simulink model "balance_bike"  (R2025a)
settings: Solver=ode45  StartTime=0.0  StopTime=50  MaxStep=0.0001  RelTol=1e-6
values from neighbouring files (symbols this model uses):
  angle_Kp = 7.5    [init_balance_bike.m]
  angle_out_max = 2000    [init_balance_bike.m]
  fly_mech_den = [J_total, B_fly]    [init_balance_bike.m]
  fly_mech_num = [1]    [init_balance_bike.m]
  gyro_Kp = 26.5    [init_balance_bike.m]
  gyro_out_max = 2000    [init_balance_bike.m]
  J_body = m_body * h_body^2    (= 0.0675)    [init_balance_bike.m]
  K_enc = PPR * Ts / (2*pi)    (= 3.18309886184)    [init_balance_bike.m]
  Ke = 0.08    [init_balance_bike.m]
  Kt = 0.08    [init_balance_bike.m]
  mgh = m_body * g * h_body    (= 4.4145)    [init_balance_bike.m]
  motor_elec_den = [La, Ra]    [init_balance_bike.m]
  motor_elec_num = [1]    [init_balance_bike.m]
  PWM_to_V = V_supply / 2000    (= 0.006)    [init_balance_bike.m]
  vel_integral_max = 500    [init_balance_bike.m]
  vel_Kd_cont = 0.015 * Ts    (= 7.5e-05)    [init_balance_bike.m]
  vel_Ki_cont = 0.000045 / Ts    (= 0.009)    [init_balance_bike.m]
  vel_Kp = 0.065    [init_balance_bike.m]
  vel_out_max = 2000    [init_balance_bike.m]
libraries: slpidlib x3
settings Model: Creator=apple  LastModifiedBy=apple

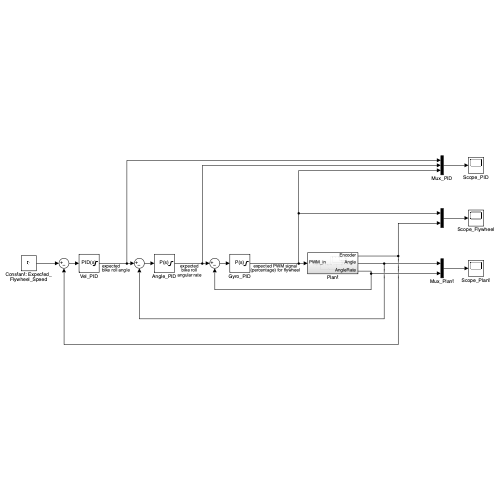
[thumbnail: Simulink's stored preview of the top-level diagram]
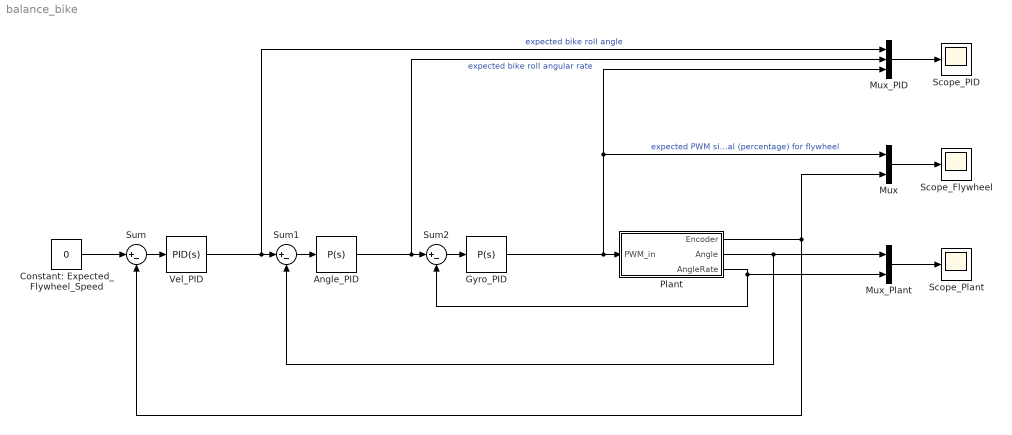
== system balance_bike ==
  Angle_PID : slpidlib/PID Controller  Controller=P  Form=Parallel  TimeDomain=Continuous-time  UseExternalTs=off  SampleTime=-1  IntegratorMethod=Forward Euler  FilterMethod=Forward Euler  ControllerParametersSource=internal  P=angle_Kp  I=1  UseKiTs=off  D=0  UseExternalDerivativeSource=off  N=100  UseFilter=on  TunerSelectOption=Transfer Function Based (PID Tuner App)  InitialConditionSource=internal  InitialConditionForIntegrator=0  InitialConditionForFilter=0  DifferentiatorICPrevScaledInput=0  ExternalReset=none  TrackingMode=off  Kt=1  LimitOutput=on  SatLimitsSource=internal  UpperSaturationLimit=angle_out_max  LowerSaturationLimit=-angle_out_max  LinearizeAsGain=on  AntiWindupMode=none  Kb=1  LimitIntegrator=off  UpperIntegratorSaturationLimit=inf  LowerIntegratorSaturationLimit=-inf  POutMin=[]  POutMax=[]  IOutMin=[]  IOutMax=[]  DOutMin=[]  DOutMax=[]  NOutMin=[]  NOutMax=[]  SumOutMin=[]  SumOutMax=[]  SaturationOutMin=[]  SaturationOutMax=[]  PParamMin=[]  PParamMax=[]  IParamMin=[]  IParamMax=[]  DParamMin=[]  DParamMax=[]  NParamMin=[]  NParamMax=[]  KbParamMin=[]  KbParamMax=[]  KtParamMin=[]  KtParamMax=[]  KbOutMin=[]  KbOutMax=[]  KtOutMin=[]  KtOutMax=[]  IntegratorOutMin=[]  IntegratorOutMax=[]  FilterOutMin=[]  FilterOutMax=[]  SumI1OutMin=[]  SumI1OutMax=[]  SumI2OutMin=[]  SumI2OutMax=[]  SumI3OutMin=[]  SumI3OutMax=[]  SumI4OutMin=[]  SumI4OutMax=[]  SumDOutMin=[]  SumDOutMax=[]  DifferentiatorOutMin=[]  DifferentiatorOutMax=[]  FilterDiffOutCoefMin=[]  FilterDiffOutCoefMax=[]  ReciprocalOutMin=[]  ReciprocalOutMax=[]  SumDenOutMin=[]  SumDenOutMax=[]  SumNumOutMin=[]  SumNumOutMax=[]  DivideOutMin=[]  DivideOutMax=[]  UdiffTsProdOutMin=[]  UdiffTsProdOutMax=[]  NTsProdOutMin=[]  NTsProdOutMax=[]  UintegralTsProdOutMin=[]  UintegralTsProdOutMax=[]  UngainTsProdOutMin=[]  UngainTsProdOutMax=[]  ClampingZeroOutDataTypeStr=Inherit: Inherit via back propagation  ClampingZeroOutMin=[]  ClampingZeroOutMax=[]  FilterDenConstantOutDataTypeStr=Inherit: Inherit via back propagation  FilterDenConstantOutMin=[]  FilterDenConstantOutMax=[]  PCopyOutDataTypeStr=Inherit: Inherit via back propagation  PCopyOutMin=[]  PCopyOutMax=[]  NCopyOutDataTypeStr=Inherit: Inherit via back propagation  NCopyOutMin=[]  NCopyOutMax=[]  IntegratorContinuousStateAttributes=''  IntegratorStateMustResolveToSignalObject=off  IntegratorRTWStateStorageClass=Auto  FilterContinuousStateAttributes=''  FilterStateMustResolveToSignalObject=off  FilterRTWStateStorageClass=Auto  ParallelPVariant=InternalParameters  IdealPVariant=Disabled  IVariant=Disabled  DVariant=Disabled  IntegratorVariant=Disabled  SatVariant=Enabled  AWVariant=Disabled  PCopyVariant=Disabled  TRVariant=Disabled  FdbkBlocksVariant=Forward  IdealPFdbkVariant=Disabled  SatFdbkVariant=Disabled  DerivativeFilterVariant=Disabled  NVariant=Disabled  NCopyVariant=Disabled_SignalSpec  FilterICVariant=Disabled  IntegratorICVariant=Disabled  ExternalResetVariant=Disabled  TRSumVariant=Passthrough  SumFdbkVariant=Disabled  SumVariant=Passthrough_P  TsampFilterVariant=InternalTs  TsampNgainVariant=Passthrough  TsampIntegralVariant=Disabled_SignalSpec  ExternalSaturationOutDataTypeStr=Inherit: Same as second input  DerivativeSourceVariant=Disabled  PreIntVariant=InternalPreInt
  Constant: Expected_ Flywheel_Speed : Constant  Value=0
  Gyro_PID : slpidlib/PID Controller  Controller=P  Form=Parallel  TimeDomain=Continuous-time  UseExternalTs=off  SampleTime=-1  IntegratorMethod=Forward Euler  FilterMethod=Forward Euler  ControllerParametersSource=internal  P=gyro_Kp  I=1  UseKiTs=off  D=0  UseExternalDerivativeSource=off  N=100  UseFilter=on  TunerSelectOption=Transfer Function Based (PID Tuner App)  InitialConditionSource=internal  InitialConditionForIntegrator=0  InitialConditionForFilter=0  DifferentiatorICPrevScaledInput=0  ExternalReset=none  TrackingMode=off  Kt=1  LimitOutput=on  SatLimitsSource=internal  UpperSaturationLimit=gyro_out_max  LowerSaturationLimit=-gyro_out_max  LinearizeAsGain=on  AntiWindupMode=none  Kb=1  LimitIntegrator=off  UpperIntegratorSaturationLimit=inf  LowerIntegratorSaturationLimit=-inf  POutMin=[]  POutMax=[]  IOutMin=[]  IOutMax=[]  DOutMin=[]  DOutMax=[]  NOutMin=[]  NOutMax=[]  SumOutMin=[]  SumOutMax=[]  SaturationOutMin=[]  SaturationOutMax=[]  PParamMin=[]  PParamMax=[]  IParamMin=[]  IParamMax=[]  DParamMin=[]  DParamMax=[]  NParamMin=[]  NParamMax=[]  KbParamMin=[]  KbParamMax=[]  KtParamMin=[]  KtParamMax=[]  KbOutMin=[]  KbOutMax=[]  KtOutMin=[]  KtOutMax=[]  IntegratorOutMin=[]  IntegratorOutMax=[]  FilterOutMin=[]  FilterOutMax=[]  SumI1OutMin=[]  SumI1OutMax=[]  SumI2OutMin=[]  SumI2OutMax=[]  SumI3OutMin=[]  SumI3OutMax=[]  SumI4OutMin=[]  SumI4OutMax=[]  SumDOutMin=[]  SumDOutMax=[]  DifferentiatorOutMin=[]  DifferentiatorOutMax=[]  FilterDiffOutCoefMin=[]  FilterDiffOutCoefMax=[]  ReciprocalOutMin=[]  ReciprocalOutMax=[]  SumDenOutMin=[]  SumDenOutMax=[]  SumNumOutMin=[]  SumNumOutMax=[]  DivideOutMin=[]  DivideOutMax=[]  UdiffTsProdOutMin=[]  UdiffTsProdOutMax=[]  NTsProdOutMin=[]  NTsProdOutMax=[]  UintegralTsProdOutMin=[]  UintegralTsProdOutMax=[]  UngainTsProdOutMin=[]  UngainTsProdOutMax=[]  ClampingZeroOutDataTypeStr=Inherit: Inherit via back propagation  ClampingZeroOutMin=[]  ClampingZeroOutMax=[]  FilterDenConstantOutDataTypeStr=Inherit: Inherit via back propagation  FilterDenConstantOutMin=[]  FilterDenConstantOutMax=[]  PCopyOutDataTypeStr=Inherit: Inherit via back propagation  PCopyOutMin=[]  PCopyOutMax=[]  NCopyOutDataTypeStr=Inherit: Inherit via back propagation  NCopyOutMin=[]  NCopyOutMax=[]  IntegratorContinuousStateAttributes=''  IntegratorStateMustResolveToSignalObject=off  IntegratorRTWStateStorageClass=Auto  FilterContinuousStateAttributes=''  FilterStateMustResolveToSignalObject=off  FilterRTWStateStorageClass=Auto  ParallelPVariant=InternalParameters  IdealPVariant=Disabled  IVariant=Disabled  DVariant=Disabled  IntegratorVariant=Disabled  SatVariant=Enabled  AWVariant=Disabled  PCopyVariant=Disabled  TRVariant=Disabled  FdbkBlocksVariant=Forward  IdealPFdbkVariant=Disabled  SatFdbkVariant=Disabled  DerivativeFilterVariant=Disabled  NVariant=Disabled  NCopyVariant=Disabled_SignalSpec  FilterICVariant=Disabled  IntegratorICVariant=Disabled  ExternalResetVariant=Disabled  TRSumVariant=Passthrough  SumFdbkVariant=Disabled  SumVariant=Passthrough_P  TsampFilterVariant=InternalTs  TsampNgainVariant=Passthrough  TsampIntegralVariant=Disabled_SignalSpec  ExternalSaturationOutDataTypeStr=Inherit: Same as second input  DerivativeSourceVariant=Disabled  PreIntVariant=InternalPreInt
  Mux : Mux  Inputs=2
  Mux_PID : Mux  Inputs=3
  Mux_Plant : Mux  Inputs=2
  Plant : Subsystem
  Scope_Flywheel : Scope
      settings: ActiveDisplayYMinimum=-2400.6327849679374  ActiveDisplayYMaximum=1605.6950647114356  DataLoggingVariableName=ScopeData3
  Scope_PID : Scope
      settings: ActiveDisplayYMinimum=-154.84030176969517  ActiveDisplayYMaximum=142.23646338458198
  Scope_Plant : Scope
      settings: ActiveDisplayYMinimum=-271.32237156661733  ActiveDisplayYMaximum=384.67484580037069  DataLoggingVariableName=ScopeData2
  Sum : Sum  Inputs=|+-
  Sum1 : Sum  Inputs=|+-
  Sum2 : Sum  Inputs=|+-
  Vel_PID : slpidlib/PID Controller  Controller=PID  Form=Parallel  TimeDomain=Continuous-time  UseExternalTs=off  SampleTime=-1  IntegratorMethod=Forward Euler  FilterMethod=Forward Euler  ControllerParametersSource=internal  P=vel_Kp  I=vel_Ki_cont  UseKiTs=off  D=vel_Kd_cont  UseExternalDerivativeSource=off  N=100  UseFilter=on  TunerSelectOption=Transfer Function Based (PID Tuner App)  InitialConditionSource=internal  InitialConditionForIntegrator=0  InitialConditionForFilter=0  DifferentiatorICPrevScaledInput=0  ExternalReset=none  TrackingMode=off  Kt=1  LimitOutput=on  SatLimitsSource=internal  UpperSaturationLimit=vel_out_max  LowerSaturationLimit=-vel_out_max  LinearizeAsGain=on  AntiWindupMode=none  Kb=1  LimitIntegrator=on  UpperIntegratorSaturationLimit=vel_integral_max  LowerIntegratorSaturationLimit=-vel_integral_max  POutMin=[]  POutMax=[]  IOutMin=[]  IOutMax=[]  DOutMin=[]  DOutMax=[]  NOutMin=[]  NOutMax=[]  SumOutMin=[]  SumOutMax=[]  SaturationOutMin=[]  SaturationOutMax=[]  PParamMin=[]  PParamMax=[]  IParamMin=[]  IParamMax=[]  DParamMin=[]  DParamMax=[]  NParamMin=[]  NParamMax=[]  KbParamMin=[]  KbParamMax=[]  KtParamMin=[]  KtParamMax=[]  KbOutMin=[]  KbOutMax=[]  KtOutMin=[]  KtOutMax=[]  IntegratorOutMin=[]  IntegratorOutMax=[]  FilterOutMin=[]  FilterOutMax=[]  SumI1OutMin=[]  SumI1OutMax=[]  SumI2OutMin=[]  SumI2OutMax=[]  SumI3OutMin=[]  SumI3OutMax=[]  SumI4OutMin=[]  SumI4OutMax=[]  SumDOutMin=[]  SumDOutMax=[]  DifferentiatorOutMin=[]  DifferentiatorOutMax=[]  FilterDiffOutCoefMin=[]  FilterDiffOutCoefMax=[]  ReciprocalOutMin=[]  ReciprocalOutMax=[]  SumDenOutMin=[]  SumDenOutMax=[]  SumNumOutMin=[]  SumNumOutMax=[]  DivideOutMin=[]  DivideOutMax=[]  UdiffTsProdOutMin=[]  UdiffTsProdOutMax=[]  NTsProdOutMin=[]  NTsProdOutMax=[]  UintegralTsProdOutMin=[]  UintegralTsProdOutMax=[]  UngainTsProdOutMin=[]  UngainTsProdOutMax=[]  ClampingZeroOutDataTypeStr=Inherit: Inherit via back propagation  ClampingZeroOutMin=[]  ClampingZeroOutMax=[]  FilterDenConstantOutDataTypeStr=Inherit: Inherit via back propagation  FilterDenConstantOutMin=[]  FilterDenConstantOutMax=[]  PCopyOutDataTypeStr=Inherit: Inherit via back propagation  PCopyOutMin=[]  PCopyOutMax=[]  NCopyOutDataTypeStr=Inherit: Inherit via back propagation  NCopyOutMin=[]  NCopyOutMax=[]  IntegratorContinuousStateAttributes=''  IntegratorStateMustResolveToSignalObject=off  IntegratorRTWStateStorageClass=Auto  FilterContinuousStateAttributes=''  FilterStateMustResolveToSignalObject=off  FilterRTWStateStorageClass=Auto  ParallelPVariant=InternalParameters  IdealPVariant=Disabled  IVariant=InternalParameters  DVariant=InternalParameters  IntegratorVariant=Continuous  SatVariant=Enabled  AWVariant=Passthrough  PCopyVariant=Disabled  TRVariant=Disabled  FdbkBlocksVariant=Forward  IdealPFdbkVariant=Disabled  SatFdbkVariant=Disabled  DerivativeFilterVariant=ContFilter  NVariant=InternalParameters  NCopyVariant=Disabled  FilterICVariant=InternalICsFilter  IntegratorICVariant=InternalICs  ExternalResetVariant=Disabled  TRSumVariant=Passthrough  SumFdbkVariant=Disabled  SumVariant=Sum_PID  TsampFilterVariant=InternalTs  TsampNgainVariant=Passthrough  TsampIntegralVariant=Disabled_SignalSpec  ExternalSaturationOutDataTypeStr=Inherit: Same as second input  DerivativeSourceVariant=ErrorSignal  PreIntVariant=InternalPreInt
  wires:
  Plant/1(Encoder) -> Mux/2, Sum/2
  Plant/3(AngleRate) -> Mux_Plant/2, Sum2/2
  Plant/2(Angle) -> Sum1/2, Mux_Plant/1
  Constant: Expected_ Flywheel_Speed/1 -> Sum/1
  Sum1/1 -> Angle_PID/1
  Sum2/1 -> Gyro_PID/1
  Angle_PID/1 -> Mux_PID/2, Sum2/1  "expected bike roll angular rate"
  Sum/1 -> Vel_PID/1
  Gyro_PID/1 -> Mux/1, Mux_PID/3, Plant/1(PWM_in)  "expected PWM signal (percentage) for flywheel"
  Mux_PID/1 -> Scope_PID/1
  Mux_Plant/1 -> Scope_Plant/1
  Vel_PID/1 -> Mux_PID/1, Sum1/1  "expected bike roll angle"
  Mux/1 -> Scope_Flywheel/1

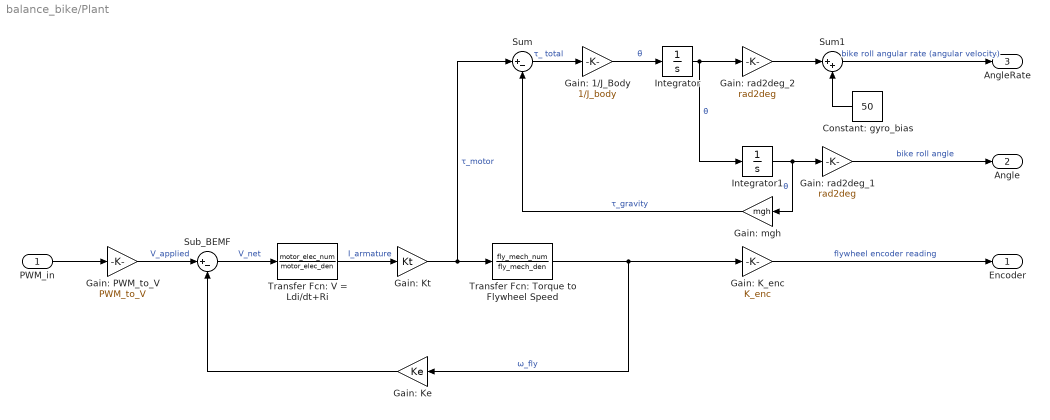
== system balance_bike/Plant ==
  PWM_in : Inport
  Constant: gyro_bias : Constant  Value=50
  Gain: 1/J_Body : Gain  Gain=1/J_body
  Gain: K_enc : Gain  Gain=K_enc
  Gain: Ke : Gain  Gain=Ke
  Gain: Kt : Gain  Gain=Kt
  Gain: PWM_to_V : Gain  Gain=PWM_to_V
  Gain: mgh : Gain  Gain=mgh
  Gain: rad2deg_1 : Gain  Gain=rad2deg
  Gain: rad2deg_2 : Gain  Gain=rad2deg
  Integrator : Integrator
  Integrator1 : Integrator  InitialCondition=0.5
  Sub_BEMF : Sum  Inputs=|+-
  Sum : Sum  Inputs=|+-
  Sum1 : Sum  Inputs=|++
  Transfer Fcn: V = Ldi/dt+Ri : TransferFcn  Numerator=motor_elec_num  Denominator=motor_elec_den
  Transfer Fcn: Torque to Flywheel Speed : TransferFcn  Numerator=fly_mech_num  Denominator=fly_mech_den
  Encoder : Outport
  Angle : Outport  Port=2
  AngleRate : Outport  Port=3
  wires:
  Gain: mgh/1 -> Sum/2  "τ_gravity"
  Gain: PWM_to_V/1 -> Sub_BEMF/1  "V_applied"
  Transfer Fcn: V = Ldi/dt+Ri/1 -> Gain: Kt/1  "I_armature"
  Integrator/1 -> Gain: rad2deg_2/1, Integrator1/1  "θ̇"
  Gain: rad2deg_2/1 -> Sum1/1
  Gain: rad2deg_1/1 -> Angle/1  "bike roll angle"
  Sum/1 -> Gain: 1/J_Body/1  "τ_ total"
  Gain: 1/J_Body/1 -> Integrator/1  "θ̈"
  Integrator1/1 -> Gain: rad2deg_1/1, Gain: mgh/1  "θ"
  Constant: gyro_bias/1 -> Sum1/2
  Gain: Kt/1 -> Sum/1, Transfer Fcn: Torque to Flywheel Speed/1  "τ_motor"
  Sub_BEMF/1 -> Transfer Fcn: V = Ldi/dt+Ri/1  "V_net"
  Gain: Ke/1 -> Sub_BEMF/2
  PWM_in/1 -> Gain: PWM_to_V/1
  Transfer Fcn: Torque to Flywheel Speed/1 -> Gain: Ke/1, Gain: K_enc/1  "ω_fly"
  Sum1/1 -> AngleRate/1  "bike roll angular rate (angular velocity)"
  Gain: K_enc/1 -> Encoder/1  "flywheel encoder reading"
